simulink model "triggered_system"  (R2017b)
settings: Solver=FixedStepDiscrete  StartTime=0.0  StopTime=10.0  RelTol=1e-3
settings Model: Creator=ibrahim  LastModifiedBy=ibrahim
settings OptimizationCC: DefaultParameterBehavior=Inlined  PassReuseOutputArgsAs=Individual arguments
settings DebuggingCC: ParameterTunabilityLossMsg=error
settings SFSimCC: MATLABDynamicMemAlloc=off
settings RTWCC: SystemTargetFile=ert.tlc  GenCodeOnly=on  TemplateMakefile=ert_default_tmf  GenerateReport=on  IncludeHyperlinkInReport=on  LaunchReport=on  GenerateTraceInfo=on  GenerateTraceReport=on  GenerateTraceReportSl=on  GenerateTraceReportSf=on  GenerateTraceReportEml=on  GenerateWebview=on
settings CodeAppCC: ForceParamTrailComments=on  IgnoreCustomStorageClasses=off  OperatorAnnotations=on  SimulinkDataObjDesc=on  SFDataObjDesc=on  InsertBlockDesc=on
settings ERTTargetCC: TargetLangStandard=C99 (ISO)  GenerateSampleERTMain=on  InlinedParameterPlacement=NonHierarchical  ERTCustomFileTemplate=example_file_process.tlc

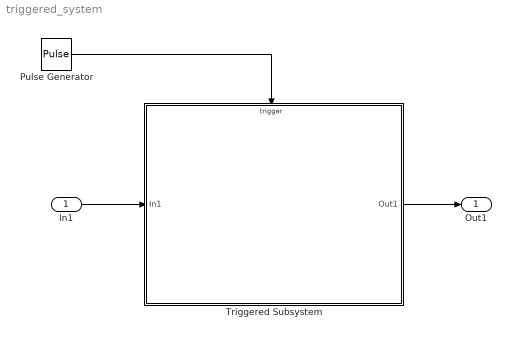
== system triggered_system ==
  In1 : Inport
  Pulse Generator : DiscretePulseGenerator  PulseType=Time based  Period=10  PulseWidth=5
  Triggered Subsystem : Subsystem  TreatAsAtomicUnit=on
  Out1 : Outport
  wires:
  In1/1 -> Triggered Subsystem/1(In1)
  Triggered Subsystem/1(Out1) -> Out1/1
  Pulse Generator/1 -> Triggered Subsystem/Trigger

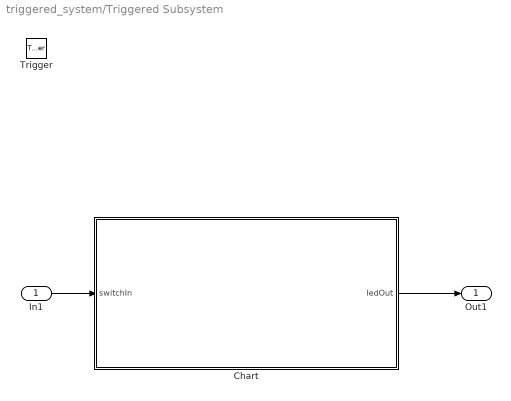
== system triggered_system/Triggered Subsystem ==
  In1 : Inport
  Trigger : TriggerPort  VariantControl=Variant
  Chart : Stateflow chart  TreatAsAtomicUnit=on
  Out1 : Outport
  wires:
  In1/1 -> Chart/1(switchIn)
  Chart/1(ledOut) -> Out1/1

== stateflow chart triggered_system/Triggered Subsystem/Chart ==
  (default) -> (junction 9) : /* check switch input */
  (junction 9) -> (junction 10) [order 1] : [switchIn == 1]
  (junction 9) -> (junction 11) [order 2] : {ledOut = 0;}
  (junction 10) -> (junction 12) : {ledOut = 1;}
  (junction 12) -> (junction 11)
  (junction 11) -> (junction 13)
  data: switchIn input; ledOut output
